simulink model "Controller"  (R2018b)
settings: configuration reference "control_config" (kept outside this file)
values from neighbouring files (symbols this model uses):
  CONTROL_EXPORT = Simulink.Parameter(CONTROL_EXPORT_VALUE)    [controller_model_init.m]
  CONTROL_PARAM = Simulink.Parameter(CONTROL_PARAM_VALUE)    [controller_model_init.m]
undefined symbols (not defined in the file or in its folder): actuator_cmd, CONTROL_CONST, CONTROL_PARAM_VALUE, ControlMode, DiscIntNeverNeededParam, PilotMode, timestamp
libraries: simulink x43, FMT_Model_Lib x6
(part 1 of 2)
settings Model: Creator=jc  LastModifiedBy=zouji
settings ConfigSetRef: SourceLocation=Base Workspace

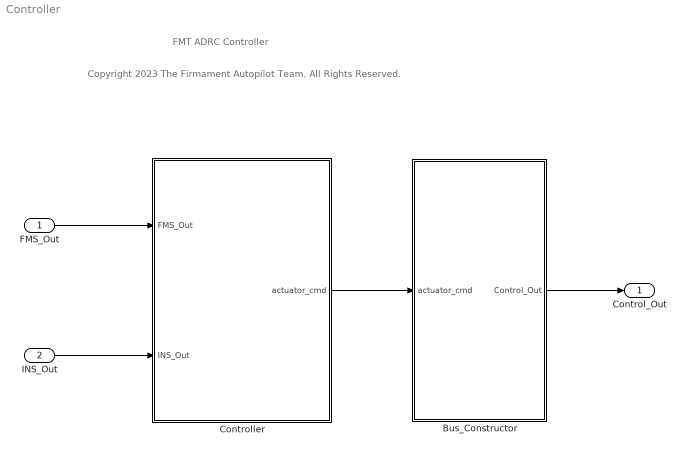
== system Controller ==
  note: Copyright 2023 The Firmament Autopilot Team. All Rights Reserved.
  note: FMT ADRC Controller
  FMS_Out : Inport  OutDataTypeStr=Bus: FMS_Out_Bus
  INS_Out : Inport  Port=2  OutDataTypeStr=Bus: INS_Out_Bus
  Bus_Constructor : Subsystem
  Controller : Subsystem
  Control_Out : Outport  OutDataTypeStr=Bus: Control_Out_Bus
  wires:
  FMS_Out/1 -> Controller/1(FMS_Out)
  INS_Out/1 -> Controller/2(INS_Out)
  Controller/1(actuator_cmd) -> Bus_Constructor/1(actuator_cmd)
  Bus_Constructor/1(Control_Out) -> Control_Out/1

== system Controller/Bus_Constructor ==
  actuator_cmd : Inport
  Bus Assignment : BusAssignment  AssignedSignals=actuator_cmd,timestamp
  Constant : Constant  Value=0  OutDataTypeStr=Bus: Control_Out_Bus
  timestamp : Subsystem  mask{sample_time=CONTROL_EXPORT.period}
      mask prompts: sample_time "sample time (ms)"
  Control_Out : Outport
  wires:
  actuator_cmd/1 -> Bus Assignment/2
  Constant/1 -> Bus Assignment/1
  Bus Assignment/1 -> Control_Out/1
  timestamp/1(timestamp_ms) -> Bus Assignment/3

== system Controller/Controller ==
  FMS_Out : Inport
  INS_Out : Inport  Port=2
  Control_Allocation : Subsystem  Variant=on
      settings: GeneratePreprocessorConditionals=on
  Horizontal_Control : Subsystem
  Vertical_Control : Subsystem
  actuator_cmd : Outport
  wires:
  FMS_Out/1 -> Control_Allocation/1(FMS_Out), Vertical_Control/1(FMS_Out), Horizontal_Control/1(FMS_Out)
  INS_Out/1 -> Horizontal_Control/2(INS_Out), Vertical_Control/2(INS_Out)
  Horizontal_Control/1(rate_dot_cmd_B) -> Control_Allocation/2(ang_acc_cmd)
  Vertical_Control/1(g_force_cmd_B) -> Control_Allocation/3(line_acc_cmd)
  Control_Allocation/1(actuator_cmd) -> actuator_cmd/1

== system Controller/Bus_Constructor/timestamp ==
  Constant : Constant  Value=sample_time
  Data Type Conversion : DataTypeConversion  OutDataTypeStr=uint32
  Discrete-Time Integrator : DiscreteIntegrator  IntegratorMethod=Accumulation: Forward Euler  SampleTime=-1  ICPrevOutput=DiscIntNeverNeededParam  ICPrevScaledInput=DiscIntNeverNeededParam
  timestamp_ms : Outport
  wires:
  Discrete-Time Integrator/1 -> Data Type Conversion/1
  Constant/1 -> Discrete-Time Integrator/1
  Data Type Conversion/1 -> timestamp_ms/1

== system Controller/Controller/Control_Allocation ==
  note: 1) Add Subsystem or Model blocks as valid variant choices.
      | 2) You cannot connect blocks at this level. At simulation, connectivity is automatically
      | determined, based on the active variant and port name matching.
  FMS_Out : Inport
  ang_acc_cmd : Inport  Port=2
  line_acc_cmd : Inport  Port=3
  Coxial_Hexacopter_x : Subsystem  TreatAsAtomicUnit=on  VariantControl=AIRFRAME==6
      mask Display: image('.\figures\cox_hexa_x.png');
  Coxial_Quadcopter_x : Subsystem  TreatAsAtomicUnit=on  VariantControl=AIRFRAME==3
      mask Display: image('.\figures\cox_quad_x.png');
  Hexacopter_+ : Subsystem  TreatAsAtomicUnit=on  VariantControl=AIRFRAME==5
      mask Display: image('.\figures\hexa_+.png');
  Hexacopter_x : Subsystem  TreatAsAtomicUnit=on  VariantControl=AIRFRAME==4
      mask Display: image('.\figures\hexa_x.png');
  Octocopter_+ : Subsystem  TreatAsAtomicUnit=on  VariantControl=AIRFRAME==8
      mask Display: image('.\figures\octo_+.png');
  Octocopter_x : Subsystem  TreatAsAtomicUnit=on  VariantControl=AIRFRAME==7
      mask Display: image('.\figures\octo_x.png');
  Quadcopter_+ : Subsystem  TreatAsAtomicUnit=on  VariantControl=AIRFRAME==2
      mask Display: image('.\figures\quad_+.png');
  Quadcopter_x : Subsystem  TreatAsAtomicUnit=on  VariantControl=AIRFRAME==1
      mask Display: image('.\figures\quad_x.png');
  actuator_cmd : Outport

== system Controller/Controller/Horizontal_Control ==
  FMS_Out : Inport
  INS_Out : Inport  Port=2
  Attitude_Controller : Subsystem
  Velocity_Controller : Subsystem
  rate_dot_cmd_B : Outport
  wires:
  Attitude_Controller/1(rate_dot_cmd_B) -> rate_dot_cmd_B/1
  FMS_Out/1 -> Attitude_Controller/2(FMS_Out), Velocity_Controller/1(FMS_Out)
  INS_Out/1 -> Velocity_Controller/2(INS_Out), Attitude_Controller/3(INS_Out)
  Velocity_Controller/1(att_cmd_B_rad) -> Attitude_Controller/1(att_cmd_B_rad)

== system Controller/Controller/Vertical_Control ==
  FMS_Out : Inport
  INS_Out : Inport  Port=2
  Veloxity_Z_Controller : Subsystem
  g_force_cmd_B : Outport
  wires:
  INS_Out/1 -> Veloxity_Z_Controller/2(INS_Out)
  Veloxity_Z_Controller/1(g_force_cmd_B) -> g_force_cmd_B/1
  FMS_Out/1 -> Veloxity_Z_Controller/1(FMS_Out)

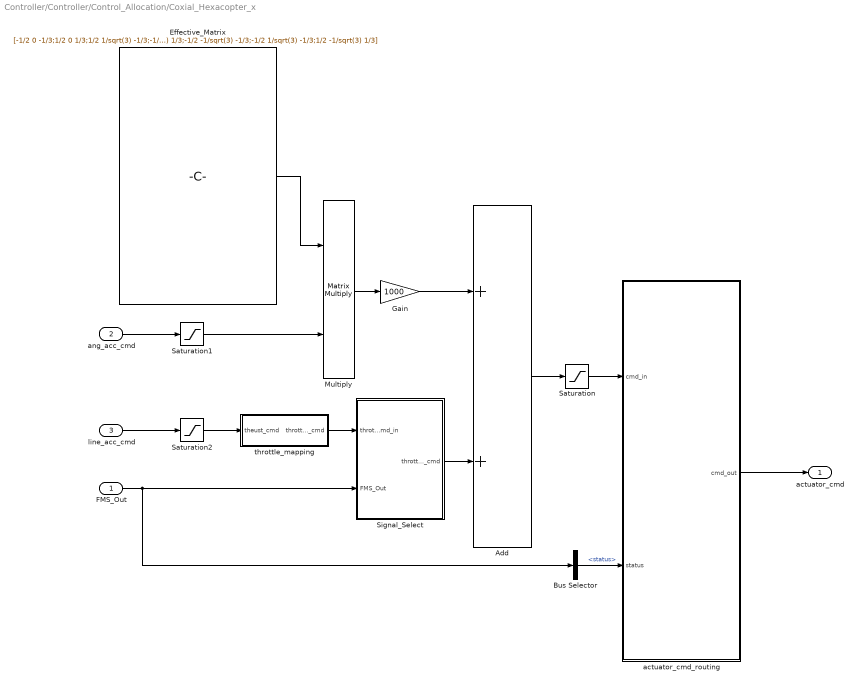
== system Controller/Controller/Control_Allocation/Coxial_Hexacopter_x ==
  FMS_Out : Inport
  ang_acc_cmd : Inport  Port=2
  line_acc_cmd : Inport  Port=3
  Add : Sum  OutDataTypeStr=uint16
  Bus Selector : BusSelector  OutputSignals=status
  Effective_Matrix : Constant  Value=[-1/2 0 -1/3;1/2 0 1/3;1/2 1/sqrt(3) -1/3;-1/2 -1/sqrt(3) 1/3;-1/2 1/sqrt(3) 1/3;1/2 -1/sqrt(3) -1/3;-1/2 0 1/3;1/2 0 -1/3;1/2 1/sqrt(3) 1/3;-1/2 -1/sqrt(3) -1/3;-1/2 1/sqrt(3) -1/3;1/2 -1/sqrt(3) 1/3]  OutDataTypeStr=single
  Gain : Gain  Gain=1000  OutDataTypeStr=uint16
  Multiply : Product  Multiplication=Matrix(*)  OutDataTypeStr=Inherit: Same as first input
  Saturation : Saturate  UpperLimit=1900  LowerLimit=1100
  Saturation1 : Saturate  UpperLimit=1  LowerLimit=-1
  Saturation2 : Saturate  UpperLimit=1  LowerLimit=-1
  Signal_Select : Subsystem
  actuator_cmd_routing : Subsystem
  throttle_mapping : Subsystem
  actuator_cmd : Outport
  wires:
  throttle_mapping/1(throttle_cmd) -> Signal_Select/1(throttle_cmd_in)
  Saturation2/1 -> throttle_mapping/1(theust_cmd)
  Gain/1 -> Add/1
  Multiply/1 -> Gain/1
  Signal_Select/1(throttle_cmd) -> Add/2
  Effective_Matrix/1 -> Multiply/1
  Saturation1/1 -> Multiply/2
  ang_acc_cmd/1 -> Saturation1/1
  line_acc_cmd/1 -> Saturation2/1
  actuator_cmd_routing/1(cmd_out) -> actuator_cmd/1
  Saturation/1 -> actuator_cmd_routing/1(cmd_in)
  FMS_Out/1 -> Bus Selector/1, Signal_Select/2(FMS_Out)
  Bus Selector/1 -> actuator_cmd_routing/2(status)  "<status>"
  Add/1 -> Saturation/1

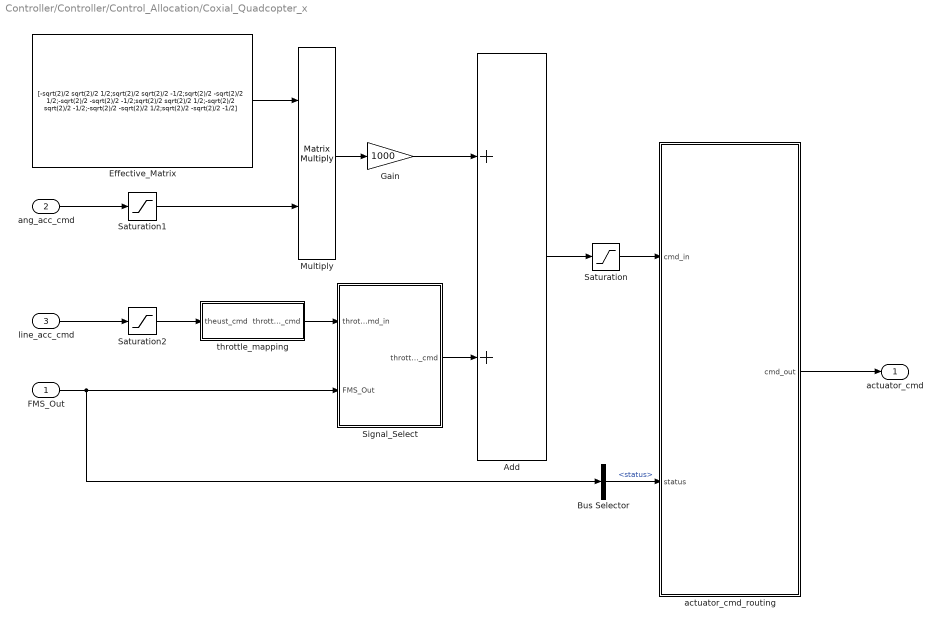
== system Controller/Controller/Control_Allocation/Coxial_Quadcopter_x ==
  FMS_Out : Inport
  ang_acc_cmd : Inport  Port=2
  line_acc_cmd : Inport  Port=3
  Add : Sum  OutDataTypeStr=uint16
  Bus Selector : BusSelector  OutputSignals=status
  Effective_Matrix : Constant  Value=[-sqrt(2)/2 sqrt(2)/2 1/2;sqrt(2)/2 sqrt(2)/2 -1/2;sqrt(2)/2 -sqrt(2)/2 1/2;-sqrt(2)/2 -sqrt(2)/2 -1/2;sqrt(2)/2 sqrt(2)/2 1/2;-sqrt(2)/2 sqrt(2)/2 -1/2;-sqrt(2)/2 -sqrt(2)/2 1/2;sqrt(2)/2 -sqrt(2)/2 -1/2]  OutDataTypeStr=single
  Gain : Gain  Gain=1000  OutDataTypeStr=uint16
  Multiply : Product  Multiplication=Matrix(*)  OutDataTypeStr=Inherit: Same as first input
  Saturation : Saturate  UpperLimit=1900  LowerLimit=1100
  Saturation1 : Saturate  UpperLimit=1  LowerLimit=-1
  Saturation2 : Saturate  UpperLimit=1  LowerLimit=-1
  Signal_Select : Subsystem
  actuator_cmd_routing : Subsystem
  throttle_mapping : Subsystem
  actuator_cmd : Outport
  wires:
  throttle_mapping/1(throttle_cmd) -> Signal_Select/1(throttle_cmd_in)
  Saturation2/1 -> throttle_mapping/1(theust_cmd)
  Gain/1 -> Add/1
  Multiply/1 -> Gain/1
  Signal_Select/1(throttle_cmd) -> Add/2
  Effective_Matrix/1 -> Multiply/1
  Saturation1/1 -> Multiply/2
  ang_acc_cmd/1 -> Saturation1/1
  line_acc_cmd/1 -> Saturation2/1
  actuator_cmd_routing/1(cmd_out) -> actuator_cmd/1
  Saturation/1 -> actuator_cmd_routing/1(cmd_in)
  FMS_Out/1 -> Bus Selector/1, Signal_Select/2(FMS_Out)
  Bus Selector/1 -> actuator_cmd_routing/2(status)  "<status>"
  Add/1 -> Saturation/1

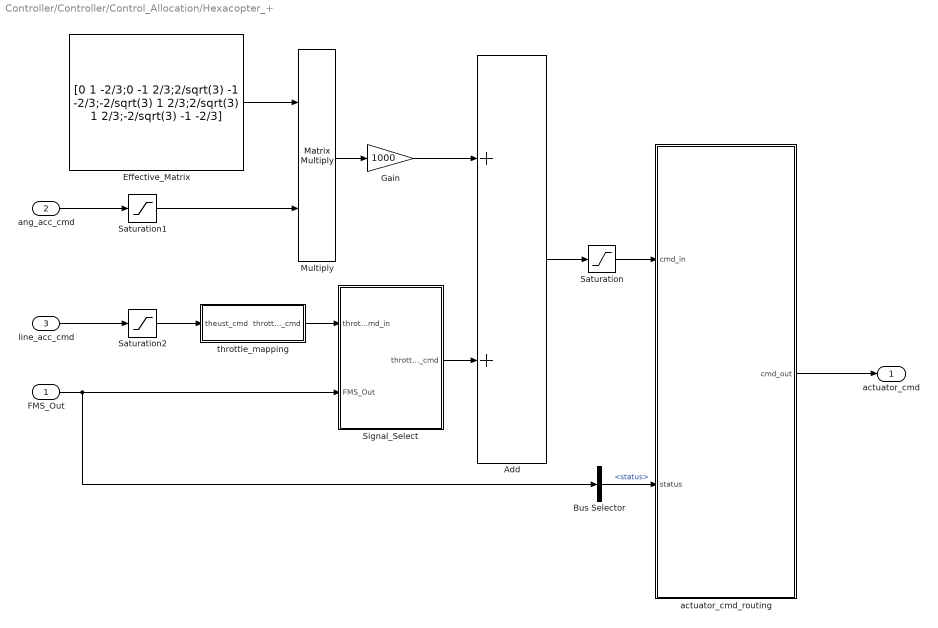
== system Controller/Controller/Control_Allocation/Hexacopter_+ ==
  FMS_Out : Inport
  ang_acc_cmd : Inport  Port=2
  line_acc_cmd : Inport  Port=3
  Add : Sum  OutDataTypeStr=uint16
  Bus Selector : BusSelector  OutputSignals=status
  Effective_Matrix : Constant  Value=[0 1 -2/3;0 -1 2/3;2/sqrt(3) -1 -2/3;-2/sqrt(3) 1 2/3;2/sqrt(3) 1 2/3;-2/sqrt(3) -1 -2/3]  OutDataTypeStr=single
  Gain : Gain  Gain=1000  OutDataTypeStr=uint16
  Multiply : Product  Multiplication=Matrix(*)  OutDataTypeStr=Inherit: Same as first input
  Saturation : Saturate  UpperLimit=1900  LowerLimit=1100
  Saturation1 : Saturate  UpperLimit=1  LowerLimit=-1
  Saturation2 : Saturate  UpperLimit=1  LowerLimit=-1
  Signal_Select : Subsystem
  actuator_cmd_routing : Subsystem
  throttle_mapping : Subsystem
  actuator_cmd : Outport
  wires:
  throttle_mapping/1(throttle_cmd) -> Signal_Select/1(throttle_cmd_in)
  Saturation2/1 -> throttle_mapping/1(theust_cmd)
  Gain/1 -> Add/1
  Multiply/1 -> Gain/1
  Signal_Select/1(throttle_cmd) -> Add/2
  Effective_Matrix/1 -> Multiply/1
  Saturation1/1 -> Multiply/2
  ang_acc_cmd/1 -> Saturation1/1
  line_acc_cmd/1 -> Saturation2/1
  actuator_cmd_routing/1(cmd_out) -> actuator_cmd/1
  Saturation/1 -> actuator_cmd_routing/1(cmd_in)
  FMS_Out/1 -> Bus Selector/1, Signal_Select/2(FMS_Out)
  Bus Selector/1 -> actuator_cmd_routing/2(status)  "<status>"
  Add/1 -> Saturation/1

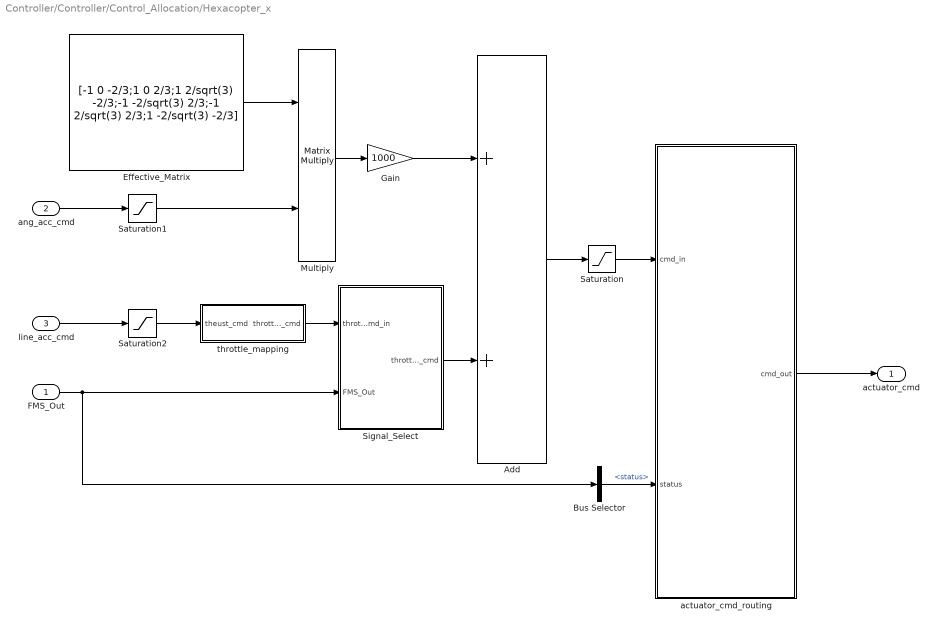
== system Controller/Controller/Control_Allocation/Hexacopter_x ==
  FMS_Out : Inport
  ang_acc_cmd : Inport  Port=2
  line_acc_cmd : Inport  Port=3
  Add : Sum  OutDataTypeStr=uint16
  Bus Selector : BusSelector  OutputSignals=status
  Effective_Matrix : Constant  Value=[-1 0 -2/3;1 0 2/3;1 2/sqrt(3) -2/3;-1 -2/sqrt(3) 2/3;-1 2/sqrt(3) 2/3;1 -2/sqrt(3) -2/3]  OutDataTypeStr=single
  Gain : Gain  Gain=1000  OutDataTypeStr=uint16
  Multiply : Product  Multiplication=Matrix(*)  OutDataTypeStr=Inherit: Same as first input
  Saturation : Saturate  UpperLimit=1900  LowerLimit=1100
  Saturation1 : Saturate  UpperLimit=1  LowerLimit=-1
  Saturation2 : Saturate  UpperLimit=1  LowerLimit=-1
  Signal_Select : Subsystem
  actuator_cmd_routing : Subsystem
  throttle_mapping : Subsystem
  actuator_cmd : Outport
  wires:
  throttle_mapping/1(throttle_cmd) -> Signal_Select/1(throttle_cmd_in)
  Saturation2/1 -> throttle_mapping/1(theust_cmd)
  Gain/1 -> Add/1
  Multiply/1 -> Gain/1
  Signal_Select/1(throttle_cmd) -> Add/2
  Effective_Matrix/1 -> Multiply/1
  Saturation1/1 -> Multiply/2
  ang_acc_cmd/1 -> Saturation1/1
  line_acc_cmd/1 -> Saturation2/1
  actuator_cmd_routing/1(cmd_out) -> actuator_cmd/1
  Saturation/1 -> actuator_cmd_routing/1(cmd_in)
  FMS_Out/1 -> Bus Selector/1, Signal_Select/2(FMS_Out)
  Bus Selector/1 -> actuator_cmd_routing/2(status)  "<status>"
  Add/1 -> Saturation/1

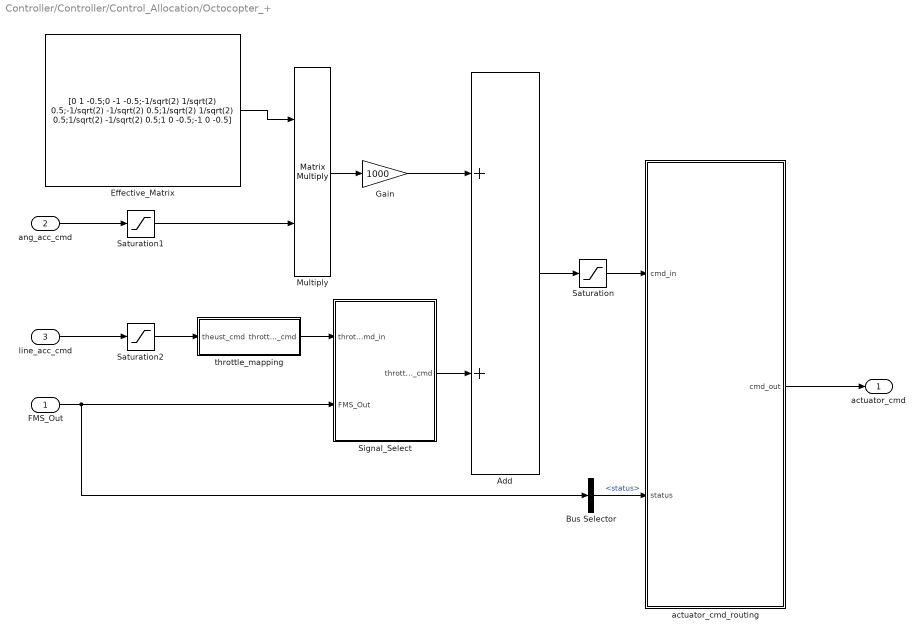
== system Controller/Controller/Control_Allocation/Octocopter_+ ==
  FMS_Out : Inport
  ang_acc_cmd : Inport  Port=2
  line_acc_cmd : Inport  Port=3
  Add : Sum  OutDataTypeStr=uint16
  Bus Selector : BusSelector  OutputSignals=status
  Effective_Matrix : Constant  Value=[0 1 -0.5;0 -1 -0.5;-1/sqrt(2) 1/sqrt(2) 0.5;-1/sqrt(2) -1/sqrt(2) 0.5;1/sqrt(2) 1/sqrt(2) 0.5;1/sqrt(2) -1/sqrt(2) 0.5;1 0 -0.5;-1 0 -0.5]  OutDataTypeStr=single
  Gain : Gain  Gain=1000  OutDataTypeStr=uint16
  Multiply : Product  Multiplication=Matrix(*)  OutDataTypeStr=Inherit: Same as first input
  Saturation : Saturate  UpperLimit=1900  LowerLimit=1100
  Saturation1 : Saturate  UpperLimit=1  LowerLimit=-1
  Saturation2 : Saturate  UpperLimit=1  LowerLimit=-1
  Signal_Select : Subsystem
  actuator_cmd_routing : Subsystem
  throttle_mapping : Subsystem
  actuator_cmd : Outport
  wires:
  throttle_mapping/1(throttle_cmd) -> Signal_Select/1(throttle_cmd_in)
  Saturation2/1 -> throttle_mapping/1(theust_cmd)
  Gain/1 -> Add/1
  Multiply/1 -> Gain/1
  Signal_Select/1(throttle_cmd) -> Add/2
  Effective_Matrix/1 -> Multiply/1
  Saturation1/1 -> Multiply/2
  ang_acc_cmd/1 -> Saturation1/1
  line_acc_cmd/1 -> Saturation2/1
  actuator_cmd_routing/1(cmd_out) -> actuator_cmd/1
  Saturation/1 -> actuator_cmd_routing/1(cmd_in)
  FMS_Out/1 -> Bus Selector/1, Signal_Select/2(FMS_Out)
  Bus Selector/1 -> actuator_cmd_routing/2(status)  "<status>"
  Add/1 -> Saturation/1

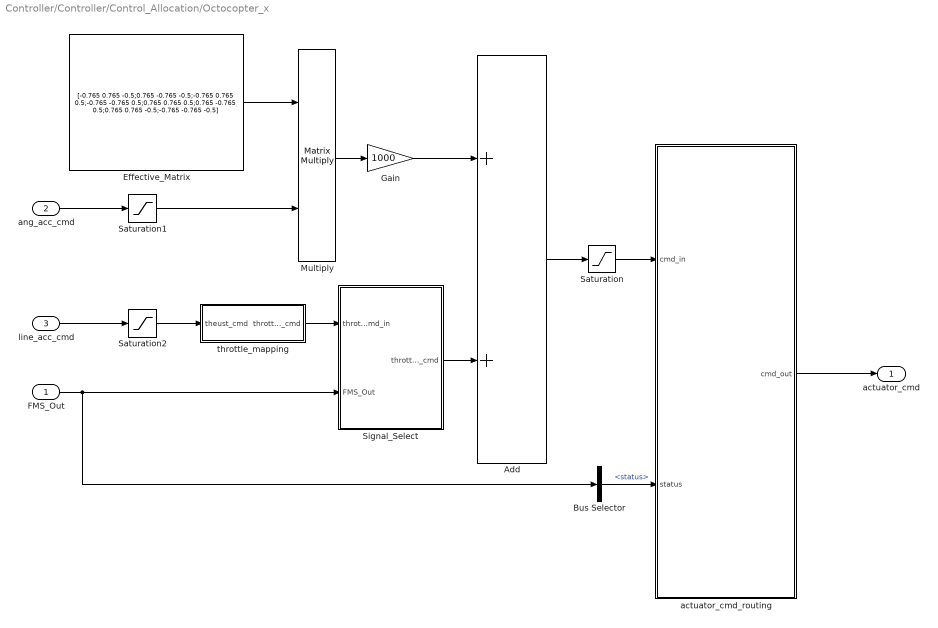
== system Controller/Controller/Control_Allocation/Octocopter_x ==
  FMS_Out : Inport
  ang_acc_cmd : Inport  Port=2
  line_acc_cmd : Inport  Port=3
  Add : Sum  OutDataTypeStr=uint16
  Bus Selector : BusSelector  OutputSignals=status
  Effective_Matrix : Constant  Value=[-0.765 0.765 -0.5;0.765 -0.765 -0.5;-0.765 0.765 0.5;-0.765 -0.765 0.5;0.765 0.765 0.5;0.765 -0.765 0.5;0.765 0.765 -0.5;-0.765 -0.765 -0.5]  OutDataTypeStr=single
  Gain : Gain  Gain=1000  OutDataTypeStr=uint16
  Multiply : Product  Multiplication=Matrix(*)  OutDataTypeStr=Inherit: Same as first input
  Saturation : Saturate  UpperLimit=1900  LowerLimit=1100
  Saturation1 : Saturate  UpperLimit=1  LowerLimit=-1
  Saturation2 : Saturate  UpperLimit=1  LowerLimit=-1
  Signal_Select : Subsystem
  actuator_cmd_routing : Subsystem
  throttle_mapping : Subsystem
  actuator_cmd : Outport
  wires:
  throttle_mapping/1(throttle_cmd) -> Signal_Select/1(throttle_cmd_in)
  Saturation2/1 -> throttle_mapping/1(theust_cmd)
  Gain/1 -> Add/1
  Multiply/1 -> Gain/1
  Signal_Select/1(throttle_cmd) -> Add/2
  Effective_Matrix/1 -> Multiply/1
  Saturation1/1 -> Multiply/2
  ang_acc_cmd/1 -> Saturation1/1
  line_acc_cmd/1 -> Saturation2/1
  actuator_cmd_routing/1(cmd_out) -> actuator_cmd/1
  Saturation/1 -> actuator_cmd_routing/1(cmd_in)
  FMS_Out/1 -> Bus Selector/1, Signal_Select/2(FMS_Out)
  Bus Selector/1 -> actuator_cmd_routing/2(status)  "<status>"
  Add/1 -> Saturation/1

== system Controller/Controller/Control_Allocation/Quadcopter_+ ==
  FMS_Out : Inport
  ang_acc_cmd : Inport  Port=2
  line_acc_cmd : Inport  Port=3
  Add : Sum  OutDataTypeStr=uint16
  Bus Selector : BusSelector  OutputSignals=status
  Effective_Matrix : Constant  Value=[-2 0 1;2 0 1;0 2 -1;0 -2 -1]  OutDataTypeStr=single
  Gain : Gain  Gain=1000  OutDataTypeStr=uint16
  Multiply : Product  Multiplication=Matrix(*)  OutDataTypeStr=Inherit: Same as first input
  Saturation : Saturate  UpperLimit=1900  LowerLimit=1100
  Saturation1 : Saturate  UpperLimit=1  LowerLimit=-1
  Saturation2 : Saturate  UpperLimit=1  LowerLimit=-1
  Signal_Select : Subsystem
  actuator_cmd_routing : Subsystem
  throttle_mapping : Subsystem
  actuator_cmd : Outport
  wires:
  throttle_mapping/1(throttle_cmd) -> Signal_Select/1(throttle_cmd_in)
  Saturation2/1 -> throttle_mapping/1(theust_cmd)
  Gain/1 -> Add/1
  Multiply/1 -> Gain/1
  Signal_Select/1(throttle_cmd) -> Add/2
  Effective_Matrix/1 -> Multiply/1
  Saturation1/1 -> Multiply/2
  ang_acc_cmd/1 -> Saturation1/1
  line_acc_cmd/1 -> Saturation2/1
  actuator_cmd_routing/1(cmd_out) -> actuator_cmd/1
  Saturation/1 -> actuator_cmd_routing/1(cmd_in)
  FMS_Out/1 -> Bus Selector/1, Signal_Select/2(FMS_Out)
  Bus Selector/1 -> actuator_cmd_routing/2(status)  "<status>"
  Add/1 -> Saturation/1

== system Controller/Controller/Control_Allocation/Quadcopter_x ==
  FMS_Out : Inport
  ang_acc_cmd : Inport  Port=2
  line_acc_cmd : Inport  Port=3
  Add : Sum  OutDataTypeStr=uint16
  Bus Selector : BusSelector  OutputSignals=status
  Effective_Matrix : Constant  Value=[-sqrt(2) sqrt(2) 1;sqrt(2) -sqrt(2) 1;sqrt(2) sqrt(2) -1;-sqrt(2) -sqrt(2) -1]  OutDataTypeStr=single
  Gain : Gain  Gain=1000  OutDataTypeStr=uint16
  Multiply : Product  Multiplication=Matrix(*)  OutDataTypeStr=Inherit: Same as first input
  Saturation : Saturate  UpperLimit=1900  LowerLimit=1100
  Saturation1 : Saturate  UpperLimit=1  LowerLimit=-1
  Saturation2 : Saturate  UpperLimit=1  LowerLimit=-1
  Signal_Select : Subsystem
  actuator_cmd_routing : Subsystem
  throttle_mapping : Subsystem
  actuator_cmd : Outport
  wires:
  throttle_mapping/1(throttle_cmd) -> Signal_Select/1(throttle_cmd_in)
  Saturation2/1 -> throttle_mapping/1(theust_cmd)
  Add/1 -> Saturation/1
  Gain/1 -> Add/1
  Multiply/1 -> Gain/1
  FMS_Out/1 -> Bus Selector/1, Signal_Select/2(FMS_Out)
  Signal_Select/1(throttle_cmd) -> Add/2
  Effective_Matrix/1 -> Multiply/1
  Saturation1/1 -> Multiply/2
  ang_acc_cmd/1 -> Saturation1/1
  line_acc_cmd/1 -> Saturation2/1
  actuator_cmd_routing/1(cmd_out) -> actuator_cmd/1
  Saturation/1 -> actuator_cmd_routing/1(cmd_in)
  Bus Selector/1 -> actuator_cmd_routing/2(status)  "<status>"

== system Controller/Controller/Horizontal_Control/Attitude_Controller ==
  att_cmd_B_rad : Inport
  FMS_Out : Inport  Port=2
  INS_Out : Inport  Port=3
  Inner_Loop : Subsystem
  Outter_Loop : Subsystem
  rate_dot_cmd_B : Outport
  wires:
  INS_Out/1 -> Inner_Loop/2(INS_Out), Outter_Loop/2(INS_Out)
  FMS_Out/1 -> Inner_Loop/3(FMS_Out), Outter_Loop/3(FMS_Out)
  att_cmd_B_rad/1 -> Outter_Loop/1(att_cmd_rad)
  Outter_Loop/1(euler_rate_cmd_radPs) -> Inner_Loop/1(euler_rate_cmd_radPs)
  Inner_Loop/1(rate_dot_cmd_B) -> rate_dot_cmd_B/1

== system Controller/Controller/Horizontal_Control/Velocity_Controller ==
  FMS_Out : Inport
  INS_Out : Inport  Port=2
  Accel_to_Attitude_CMD : Subsystem
  Bus Selector : BusSelector  OutputSignals=reset
  Error : Subsystem
  PID_Controller : Subsystem
  Signal_Select : Subsystem
  att_cmd_B_rad : Outport
  wires:
  FMS_Out/1 -> Error/2(FMS_Out), Signal_Select/2(FMS_Out), Bus Selector/1
  PID_Controller/1(accel_cmd_C) -> Signal_Select/1(acc_cmd_in)  "accel_cmd_C_mPs2"
  INS_Out/1 -> Error/1(INS_Out)
  Error/1(uv_err_C_mPs) -> PID_Controller/1(uv_err_C_mPs)
  Accel_to_Attitude_CMD/1(att_cmd_B_rad) -> att_cmd_B_rad/1
  Bus Selector/1 -> PID_Controller/2(reset)  "<reset>"
  Signal_Select/1(acc_cmd_out) -> Accel_to_Attitude_CMD/1(accel_cmd_C_mPs2)

== system Controller/Controller/Vertical_Control/Veloxity_Z_Controller ==
  note: Leave some margin
      | for att control
  FMS_Out : Inport
  INS_Out : Inport  Port=2
  Boosted_Throttle : Subsystem
  Bus Selector : BusSelector  OutputSignals=reset
  Error : Subsystem
  PID_Controller : Subsystem
  Saturation : Saturate  UpperLimit=0.35  LowerLimit=-0.35
  g_force_cmd_B : Outport
  wires:
  Saturation/1 -> g_force_cmd_B/1
  FMS_Out/1 -> Error/1(FMS_Out), Bus Selector/1
  INS_Out/1 -> Error/2(INS_Out), Boosted_Throttle/2(INS_Out)
  Boosted_Throttle/1(boosted_thrust) -> Saturation/1  "boosted_thrust"
  Error/1(az_cmd_C_mPs2) -> PID_Controller/1(az_cmd_C_mPs2)
  Bus Selector/1 -> PID_Controller/2(reset)  "<reset>"
  PID_Controller/1(thrust_cmd) -> Boosted_Throttle/1(thrust_cmd)

== system Controller/Controller/Control_Allocation/Coxial_Hexacopter_x/Signal_Select ==
  note: mode:
      | 0: Unknown
      | 1: Mission
      | 2: Position
      | 3: Altitude Hold
      | 4: Manual Mode
      | 5: Acro Mode
  throttle_cmd_in : Inport
  FMS_Out : Inport  Port=2
  Bus Selector1 : BusSelector  OutputSignals=throttle_cmd,ctrl_mode
  Compare To Constant : simulink/Logic and Bit Operations/Compare To Constant  relop===  const=uint8([ControlMode.Manual, ControlMode.Acro, ControlMode.Stabilize])  OutDataTypeStr=boolean
  Compare To Constant1 : simulink/Logic and Bit Operations/Compare To Constant  relop===  const=uint8(ControlMode.Offboard)  OutDataTypeStr=boolean
  Logical Operator : Logic  Operator=OR  Inputs=1  AllPortsSameDT=off  OutDataTypeStr=boolean
  Offboard_Signal_Select : Subsystem
  Switch : Switch  Criteria=u2 > Threshold
  Switch1 : Switch  Criteria=u2 > Threshold
  throttle_cmd : Outport
  wires:
  Compare To Constant/1 -> Logical Operator/1
  FMS_Out/1 -> Offboard_Signal_Select/1(FMS_Out), Bus Selector1/1
  Bus Selector1/1 -> Switch/1  "<throttle_cmd>"
  Bus Selector1/2 -> Compare To Constant1/1, Compare To Constant/1  "<ctrl_mode>"
  Switch/1 -> throttle_cmd/1  "throttle_cmd"
  Logical Operator/1 -> Switch/2
  throttle_cmd_in/1 -> Offboard_Signal_Select/2(throttle_cmd_in), Switch1/3
  Compare To Constant1/1 -> Switch1/2
  Switch1/1 -> Switch/3
  Offboard_Signal_Select/1(throttle_cmd_out) -> Switch1/1

== system Controller/Controller/Control_Allocation/Coxial_Hexacopter_x/actuator_cmd_routing ==
  cmd_in : Inport
  status : Inport  Port=2
  Constant : Constant  Value=zeros(4,1)  VectorParams1D=off  OutDataTypeStr=uint16
  Disarm : Constant  Value=ones(12,1)*1000  VectorParams1D=off  OutDataTypeStr=uint16
  Multiport Switch : MultiPortSwitch  DataPortForDefault=Additional data port  DiagnosticForDefault=None
  Mux1 : Mux  Inputs=2
  Reshape : Reshape  OutputDimensionality=Customize  OutputDimensions=[16,1]
  Standby : Constant  Value=ones(12,1)*1150  VectorParams1D=off  OutDataTypeStr=uint16
  cmd_out : Outport
  wires:
  Disarm/1 -> Multiport Switch/5, Multiport Switch/2
  Reshape/1 -> cmd_out/1
  Constant/1 -> Mux1/2
  Standby/1 -> Multiport Switch/3
  Mux1/1 -> Reshape/1
  status/1 -> Multiport Switch/1
  Multiport Switch/1 -> Mux1/1
  cmd_in/1 -> Multiport Switch/4

== system Controller/Controller/Control_Allocation/Coxial_Hexacopter_x/throttle_mapping ==
  theust_cmd : Inport
  Constant1 : Constant  Value=1000  OutDataTypeStr=uint32
  Data Type Conversion : DataTypeConversion  OutDataTypeStr=uint16
  Gain1 : Gain  Gain=1000  OutDataTypeStr=uint32
  Saturation : Saturate  UpperLimit=1  LowerLimit=0
  Sum : Sum  Inputs=|++
  Sum1 : Sum  Inputs=|++
  hover_throttle : Constant  Value=CONTROL_PARAM.HOVER_THRO  OutDataTypeStr=Inherit: Inherit via back propagation
  throttle_cmd : Outport
  wires:
  theust_cmd/1 -> Sum/1
  Sum/1 -> Saturation/1
  hover_throttle/1 -> Sum/2
  Gain1/1 -> Sum1/1
  Constant1/1 -> Sum1/2
  Data Type Conversion/1 -> throttle_cmd/1
  Saturation/1 -> Gain1/1
  Sum1/1 -> Data Type Conversion/1

== system Controller/Controller/Control_Allocation/Coxial_Quadcopter_x/Signal_Select ==
  note: mode:
      | 0: Unknown
      | 1: Mission
      | 2: Position
      | 3: Altitude Hold
      | 4: Manual Mode
      | 5: Acro Mode
  throttle_cmd_in : Inport
  FMS_Out : Inport  Port=2
  Bus Selector1 : BusSelector  OutputSignals=throttle_cmd,ctrl_mode
  Compare To Constant : simulink/Logic and Bit Operations/Compare To Constant  relop===  const=uint8([ControlMode.Manual, ControlMode.Acro, ControlMode.Stabilize])  OutDataTypeStr=boolean
  Compare To Constant1 : simulink/Logic and Bit Operations/Compare To Constant  relop===  const=uint8(ControlMode.Offboard)  OutDataTypeStr=boolean
  Logical Operator : Logic  Operator=OR  Inputs=1  AllPortsSameDT=off  OutDataTypeStr=boolean
  Offboard_Signal_Select : Subsystem
  Switch : Switch  Criteria=u2 > Threshold
  Switch1 : Switch  Criteria=u2 > Threshold
  throttle_cmd : Outport
  wires:
  Compare To Constant/1 -> Logical Operator/1
  FMS_Out/1 -> Offboard_Signal_Select/1(FMS_Out), Bus Selector1/1
  Bus Selector1/1 -> Switch/1  "<throttle_cmd>"
  Bus Selector1/2 -> Compare To Constant1/1, Compare To Constant/1  "<ctrl_mode>"
  Switch/1 -> throttle_cmd/1  "throttle_cmd"
  Logical Operator/1 -> Switch/2
  throttle_cmd_in/1 -> Offboard_Signal_Select/2(throttle_cmd_in), Switch1/3
  Compare To Constant1/1 -> Switch1/2
  Switch1/1 -> Switch/3
  Offboard_Signal_Select/1(throttle_cmd_out) -> Switch1/1

== system Controller/Controller/Control_Allocation/Coxial_Quadcopter_x/actuator_cmd_routing ==
  cmd_in : Inport
  status : Inport  Port=2
  Constant : Constant  Value=zeros(8,1)  VectorParams1D=off  OutDataTypeStr=uint16
  Disarm : Constant  Value=ones(8,1)*1000  VectorParams1D=off  OutDataTypeStr=uint16
  Multiport Switch : MultiPortSwitch  DataPortForDefault=Additional data port  DiagnosticForDefault=None
  Mux1 : Mux  Inputs=2
  Reshape : Reshape  OutputDimensionality=Customize  OutputDimensions=[16,1]
  Standby : Constant  Value=ones(8,1)*1150  VectorParams1D=off  OutDataTypeStr=uint16
  cmd_out : Outport
  wires:
  Disarm/1 -> Multiport Switch/5, Multiport Switch/2
  Reshape/1 -> cmd_out/1
  Constant/1 -> Mux1/2
  Standby/1 -> Multiport Switch/3
  Mux1/1 -> Reshape/1
  status/1 -> Multiport Switch/1
  Multiport Switch/1 -> Mux1/1
  cmd_in/1 -> Multiport Switch/4

== system Controller/Controller/Control_Allocation/Coxial_Quadcopter_x/throttle_mapping ==
  theust_cmd : Inport
  Constant1 : Constant  Value=1000  OutDataTypeStr=uint32
  Data Type Conversion : DataTypeConversion  OutDataTypeStr=uint16
  Gain1 : Gain  Gain=1000  OutDataTypeStr=uint32
  Saturation : Saturate  UpperLimit=1  LowerLimit=0
  Sum : Sum  Inputs=|++
  Sum1 : Sum  Inputs=|++
  hover_throttle : Constant  Value=CONTROL_PARAM.HOVER_THRO  OutDataTypeStr=Inherit: Inherit via back propagation
  throttle_cmd : Outport
  wires:
  theust_cmd/1 -> Sum/1
  Sum/1 -> Saturation/1
  hover_throttle/1 -> Sum/2
  Gain1/1 -> Sum1/1
  Constant1/1 -> Sum1/2
  Data Type Conversion/1 -> throttle_cmd/1
  Saturation/1 -> Gain1/1
  Sum1/1 -> Data Type Conversion/1

== system Controller/Controller/Control_Allocation/Hexacopter_+/Signal_Select ==
  note: mode:
      | 0: Unknown
      | 1: Mission
      | 2: Position
      | 3: Altitude Hold
      | 4: Manual Mode
      | 5: Acro Mode
  throttle_cmd_in : Inport
  FMS_Out : Inport  Port=2
  Bus Selector1 : BusSelector  OutputSignals=throttle_cmd,ctrl_mode
  Compare To Constant : simulink/Logic and Bit Operations/Compare To Constant  relop===  const=uint8([ControlMode.Manual, ControlMode.Acro, ControlMode.Stabilize])  OutDataTypeStr=boolean
  Compare To Constant1 : simulink/Logic and Bit Operations/Compare To Constant  relop===  const=uint8(ControlMode.Offboard)  OutDataTypeStr=boolean
  Logical Operator : Logic  Operator=OR  Inputs=1  AllPortsSameDT=off  OutDataTypeStr=boolean
  Offboard_Signal_Select : Subsystem
  Switch : Switch  Criteria=u2 > Threshold
  Switch1 : Switch  Criteria=u2 > Threshold
  throttle_cmd : Outport
  wires:
  Compare To Constant/1 -> Logical Operator/1
  FMS_Out/1 -> Offboard_Signal_Select/1(FMS_Out), Bus Selector1/1
  Bus Selector1/1 -> Switch/1  "<throttle_cmd>"
  Bus Selector1/2 -> Compare To Constant1/1, Compare To Constant/1  "<ctrl_mode>"
  Switch/1 -> throttle_cmd/1  "throttle_cmd"
  Logical Operator/1 -> Switch/2
  throttle_cmd_in/1 -> Offboard_Signal_Select/2(throttle_cmd_in), Switch1/3
  Compare To Constant1/1 -> Switch1/2
  Switch1/1 -> Switch/3
  Offboard_Signal_Select/1(throttle_cmd_out) -> Switch1/1

== system Controller/Controller/Control_Allocation/Hexacopter_+/actuator_cmd_routing ==
  cmd_in : Inport
  status : Inport  Port=2
  Constant : Constant  Value=zeros(10,1)  VectorParams1D=off  OutDataTypeStr=uint16
  Disarm : Constant  Value=ones(6,1)*1000  VectorParams1D=off  OutDataTypeStr=uint16
  Multiport Switch : MultiPortSwitch  DataPortForDefault=Additional data port  DiagnosticForDefault=None
  Mux1 : Mux  Inputs=2
  Reshape : Reshape  OutputDimensionality=Customize  OutputDimensions=[16,1]
  Standby : Constant  Value=ones(6,1)*1150  VectorParams1D=off  OutDataTypeStr=uint16
  cmd_out : Outport
  wires:
  Disarm/1 -> Multiport Switch/5, Multiport Switch/2
  Reshape/1 -> cmd_out/1
  Constant/1 -> Mux1/2
  Standby/1 -> Multiport Switch/3
  Mux1/1 -> Reshape/1
  status/1 -> Multiport Switch/1
  Multiport Switch/1 -> Mux1/1
  cmd_in/1 -> Multiport Switch/4

== system Controller/Controller/Control_Allocation/Hexacopter_+/throttle_mapping ==
  theust_cmd : Inport
  Constant1 : Constant  Value=1000  OutDataTypeStr=uint32
  Data Type Conversion : DataTypeConversion  OutDataTypeStr=uint16
  Gain1 : Gain  Gain=1000  OutDataTypeStr=uint32
  Saturation : Saturate  UpperLimit=1  LowerLimit=0
  Sum : Sum  Inputs=|++
  Sum1 : Sum  Inputs=|++
  hover_throttle : Constant  Value=CONTROL_PARAM.HOVER_THRO  OutDataTypeStr=Inherit: Inherit via back propagation
  throttle_cmd : Outport
  wires:
  theust_cmd/1 -> Sum/1
  Sum/1 -> Saturation/1
  hover_throttle/1 -> Sum/2
  Gain1/1 -> Sum1/1
  Constant1/1 -> Sum1/2
  Data Type Conversion/1 -> throttle_cmd/1
  Saturation/1 -> Gain1/1
  Sum1/1 -> Data Type Conversion/1

== system Controller/Controller/Control_Allocation/Hexacopter_x/Signal_Select ==
  note: mode:
      | 0: Unknown
      | 1: Mission
      | 2: Position
      | 3: Altitude Hold
      | 4: Manual Mode
      | 5: Acro Mode
  throttle_cmd_in : Inport
  FMS_Out : Inport  Port=2
  Bus Selector1 : BusSelector  OutputSignals=throttle_cmd,ctrl_mode
  Compare To Constant : simulink/Logic and Bit Operations/Compare To Constant  relop===  const=uint8([ControlMode.Manual, ControlMode.Acro, ControlMode.Stabilize])  OutDataTypeStr=boolean
  Compare To Constant1 : simulink/Logic and Bit Operations/Compare To Constant  relop===  const=uint8(ControlMode.Offboard)  OutDataTypeStr=boolean
  Logical Operator : Logic  Operator=OR  Inputs=1  AllPortsSameDT=off  OutDataTypeStr=boolean
  Offboard_Signal_Select : Subsystem
  Switch : Switch  Criteria=u2 > Threshold
  Switch1 : Switch  Criteria=u2 > Threshold
  throttle_cmd : Outport
  wires:
  Compare To Constant/1 -> Logical Operator/1
  FMS_Out/1 -> Offboard_Signal_Select/1(FMS_Out), Bus Selector1/1
  Bus Selector1/1 -> Switch/1  "<throttle_cmd>"
  Bus Selector1/2 -> Compare To Constant1/1, Compare To Constant/1  "<ctrl_mode>"
  Switch/1 -> throttle_cmd/1  "throttle_cmd"
  Logical Operator/1 -> Switch/2
  throttle_cmd_in/1 -> Offboard_Signal_Select/2(throttle_cmd_in), Switch1/3
  Compare To Constant1/1 -> Switch1/2
  Switch1/1 -> Switch/3
  Offboard_Signal_Select/1(throttle_cmd_out) -> Switch1/1

== system Controller/Controller/Control_Allocation/Hexacopter_x/actuator_cmd_routing ==
  cmd_in : Inport
  status : Inport  Port=2
  Constant : Constant  Value=zeros(10,1)  VectorParams1D=off  OutDataTypeStr=uint16
  Disarm : Constant  Value=ones(6,1)*1000  VectorParams1D=off  OutDataTypeStr=uint16
  Multiport Switch : MultiPortSwitch  DataPortForDefault=Additional data port  DiagnosticForDefault=None
  Mux1 : Mux  Inputs=2
  Reshape : Reshape  OutputDimensionality=Customize  OutputDimensions=[16,1]
  Standby : Constant  Value=ones(6,1)*1150  VectorParams1D=off  OutDataTypeStr=uint16
  cmd_out : Outport
  wires:
  Disarm/1 -> Multiport Switch/5, Multiport Switch/2
  Reshape/1 -> cmd_out/1
  Constant/1 -> Mux1/2
  Standby/1 -> Multiport Switch/3
  Mux1/1 -> Reshape/1
  status/1 -> Multiport Switch/1
  Multiport Switch/1 -> Mux1/1
  cmd_in/1 -> Multiport Switch/4

== system Controller/Controller/Control_Allocation/Hexacopter_x/throttle_mapping ==
  theust_cmd : Inport
  Constant1 : Constant  Value=1000  OutDataTypeStr=uint32
  Data Type Conversion : DataTypeConversion  OutDataTypeStr=uint16
  Gain1 : Gain  Gain=1000  OutDataTypeStr=uint32
  Saturation : Saturate  UpperLimit=1  LowerLimit=0
  Sum : Sum  Inputs=|++
  Sum1 : Sum  Inputs=|++
  hover_throttle : Constant  Value=CONTROL_PARAM.HOVER_THRO  OutDataTypeStr=Inherit: Inherit via back propagation
  throttle_cmd : Outport
  wires:
  theust_cmd/1 -> Sum/1
  Sum/1 -> Saturation/1
  hover_throttle/1 -> Sum/2
  Gain1/1 -> Sum1/1
  Constant1/1 -> Sum1/2
  Data Type Conversion/1 -> throttle_cmd/1
  Saturation/1 -> Gain1/1
  Sum1/1 -> Data Type Conversion/1

== system Controller/Controller/Control_Allocation/Octocopter_+/Signal_Select ==
  note: mode:
      | 0: Unknown
      | 1: Mission
      | 2: Position
      | 3: Altitude Hold
      | 4: Manual Mode
      | 5: Acro Mode
  throttle_cmd_in : Inport
  FMS_Out : Inport  Port=2
  Bus Selector1 : BusSelector  OutputSignals=throttle_cmd,ctrl_mode
  Compare To Constant : simulink/Logic and Bit Operations/Compare To Constant  relop===  const=uint8([ControlMode.Manual, ControlMode.Acro, ControlMode.Stabilize])  OutDataTypeStr=boolean
  Compare To Constant1 : simulink/Logic and Bit Operations/Compare To Constant  relop===  const=uint8(ControlMode.Offboard)  OutDataTypeStr=boolean
  Logical Operator : Logic  Operator=OR  Inputs=1  AllPortsSameDT=off  OutDataTypeStr=boolean
  Offboard_Signal_Select : Subsystem
  Switch : Switch  Criteria=u2 > Threshold
  Switch1 : Switch  Criteria=u2 > Threshold
  throttle_cmd : Outport
  wires:
  Compare To Constant/1 -> Logical Operator/1
  FMS_Out/1 -> Offboard_Signal_Select/1(FMS_Out), Bus Selector1/1
  Bus Selector1/1 -> Switch/1  "<throttle_cmd>"
  Bus Selector1/2 -> Compare To Constant1/1, Compare To Constant/1  "<ctrl_mode>"
  Switch/1 -> throttle_cmd/1  "throttle_cmd"
  Logical Operator/1 -> Switch/2
  throttle_cmd_in/1 -> Offboard_Signal_Select/2(throttle_cmd_in), Switch1/3
  Compare To Constant1/1 -> Switch1/2
  Switch1/1 -> Switch/3
  Offboard_Signal_Select/1(throttle_cmd_out) -> Switch1/1

== system Controller/Controller/Control_Allocation/Octocopter_+/actuator_cmd_routing ==
  cmd_in : Inport
  status : Inport  Port=2
  Constant : Constant  Value=zeros(8,1)  VectorParams1D=off  OutDataTypeStr=uint16
  Disarm : Constant  Value=ones(8,1)*1000  VectorParams1D=off  OutDataTypeStr=uint16
  Multiport Switch : MultiPortSwitch  DataPortForDefault=Additional data port  DiagnosticForDefault=None
  Mux1 : Mux  Inputs=2
  Reshape : Reshape  OutputDimensionality=Customize  OutputDimensions=[16,1]
  Standby : Constant  Value=ones(8,1)*1150  VectorParams1D=off  OutDataTypeStr=uint16
  cmd_out : Outport
  wires:
  Disarm/1 -> Multiport Switch/5, Multiport Switch/2
  Reshape/1 -> cmd_out/1
  Constant/1 -> Mux1/2
  Standby/1 -> Multiport Switch/3
  Mux1/1 -> Reshape/1
  status/1 -> Multiport Switch/1
  Multiport Switch/1 -> Mux1/1
  cmd_in/1 -> Multiport Switch/4

== system Controller/Controller/Control_Allocation/Octocopter_+/throttle_mapping ==
  theust_cmd : Inport
  Constant1 : Constant  Value=1000  OutDataTypeStr=uint32
  Data Type Conversion : DataTypeConversion  OutDataTypeStr=uint16
  Gain1 : Gain  Gain=1000  OutDataTypeStr=uint32
  Saturation : Saturate  UpperLimit=1  LowerLimit=0
  Sum : Sum  Inputs=|++
  Sum1 : Sum  Inputs=|++
  hover_throttle : Constant  Value=CONTROL_PARAM.HOVER_THRO  OutDataTypeStr=Inherit: Inherit via back propagation
  throttle_cmd : Outport
  wires:
  theust_cmd/1 -> Sum/1
  Sum/1 -> Saturation/1
  hover_throttle/1 -> Sum/2
  Gain1/1 -> Sum1/1
  Constant1/1 -> Sum1/2
  Data Type Conversion/1 -> throttle_cmd/1
  Saturation/1 -> Gain1/1
  Sum1/1 -> Data Type Conversion/1

== system Controller/Controller/Control_Allocation/Octocopter_x/Signal_Select ==
  note: mode:
      | 0: Unknown
      | 1: Mission
      | 2: Position
      | 3: Altitude Hold
      | 4: Manual Mode
      | 5: Acro Mode
  throttle_cmd_in : Inport
  FMS_Out : Inport  Port=2
  Bus Selector1 : BusSelector  OutputSignals=throttle_cmd,ctrl_mode
  Compare To Constant : simulink/Logic and Bit Operations/Compare To Constant  relop===  const=uint8([ControlMode.Manual, ControlMode.Acro, ControlMode.Stabilize])  OutDataTypeStr=boolean
  Compare To Constant1 : simulink/Logic and Bit Operations/Compare To Constant  relop===  const=uint8(ControlMode.Offboard)  OutDataTypeStr=boolean
  Logical Operator : Logic  Operator=OR  Inputs=1  AllPortsSameDT=off  OutDataTypeStr=boolean
  Offboard_Signal_Select : Subsystem
  Switch : Switch  Criteria=u2 > Threshold
  Switch1 : Switch  Criteria=u2 > Threshold
  throttle_cmd : Outport
  wires:
  Compare To Constant/1 -> Logical Operator/1
  FMS_Out/1 -> Offboard_Signal_Select/1(FMS_Out), Bus Selector1/1
  Bus Selector1/1 -> Switch/1  "<throttle_cmd>"
  Bus Selector1/2 -> Compare To Constant1/1, Compare To Constant/1  "<ctrl_mode>"
  Switch/1 -> throttle_cmd/1  "throttle_cmd"
  Logical Operator/1 -> Switch/2
  throttle_cmd_in/1 -> Offboard_Signal_Select/2(throttle_cmd_in), Switch1/3
  Compare To Constant1/1 -> Switch1/2
  Switch1/1 -> Switch/3
  Offboard_Signal_Select/1(throttle_cmd_out) -> Switch1/1

== system Controller/Controller/Control_Allocation/Octocopter_x/actuator_cmd_routing ==
  cmd_in : Inport
  status : Inport  Port=2
  Constant : Constant  Value=zeros(8,1)  VectorParams1D=off  OutDataTypeStr=uint16
  Disarm : Constant  Value=ones(8,1)*1000  VectorParams1D=off  OutDataTypeStr=uint16
  Multiport Switch : MultiPortSwitch  DataPortForDefault=Additional data port  DiagnosticForDefault=None
  Mux1 : Mux  Inputs=2
  Reshape : Reshape  OutputDimensionality=Customize  OutputDimensions=[16,1]
  Standby : Constant  Value=ones(8,1)*1150  VectorParams1D=off  OutDataTypeStr=uint16
  cmd_out : Outport
  wires:
  Disarm/1 -> Multiport Switch/5, Multiport Switch/2
  Reshape/1 -> cmd_out/1
  Constant/1 -> Mux1/2
  Standby/1 -> Multiport Switch/3
  Mux1/1 -> Reshape/1
  status/1 -> Multiport Switch/1
  Multiport Switch/1 -> Mux1/1
  cmd_in/1 -> Multiport Switch/4

== system Controller/Controller/Control_Allocation/Octocopter_x/throttle_mapping ==
  theust_cmd : Inport
  Constant1 : Constant  Value=1000  OutDataTypeStr=uint32
  Data Type Conversion : DataTypeConversion  OutDataTypeStr=uint16
  Gain1 : Gain  Gain=1000  OutDataTypeStr=uint32
  Saturation : Saturate  UpperLimit=1  LowerLimit=0
  Sum : Sum  Inputs=|++
  Sum1 : Sum  Inputs=|++
  hover_throttle : Constant  Value=CONTROL_PARAM.HOVER_THRO  OutDataTypeStr=Inherit: Inherit via back propagation
  throttle_cmd : Outport
  wires:
  theust_cmd/1 -> Sum/1
  Sum/1 -> Saturation/1
  hover_throttle/1 -> Sum/2
  Gain1/1 -> Sum1/1
  Constant1/1 -> Sum1/2
  Data Type Conversion/1 -> throttle_cmd/1
  Saturation/1 -> Gain1/1
  Sum1/1 -> Data Type Conversion/1

== system Controller/Controller/Control_Allocation/Quadcopter_+/Signal_Select ==
  note: mode:
      | 0: Unknown
      | 1: Mission
      | 2: Position
      | 3: Altitude Hold
      | 4: Manual Mode
      | 5: Acro Mode
  throttle_cmd_in : Inport
  FMS_Out : Inport  Port=2
  Bus Selector1 : BusSelector  OutputSignals=throttle_cmd,ctrl_mode
  Compare To Constant : simulink/Logic and Bit Operations/Compare To Constant  relop===  const=uint8([ControlMode.Manual, ControlMode.Acro, ControlMode.Stabilize])  OutDataTypeStr=boolean
  Compare To Constant1 : simulink/Logic and Bit Operations/Compare To Constant  relop===  const=uint8(ControlMode.Offboard)  OutDataTypeStr=boolean
  Logical Operator : Logic  Operator=OR  Inputs=1  AllPortsSameDT=off  OutDataTypeStr=boolean
  Offboard_Signal_Select : Subsystem
  Switch : Switch  Criteria=u2 > Threshold
  Switch1 : Switch  Criteria=u2 > Threshold
  throttle_cmd : Outport
  wires:
  Compare To Constant/1 -> Logical Operator/1
  FMS_Out/1 -> Offboard_Signal_Select/1(FMS_Out), Bus Selector1/1
  Bus Selector1/1 -> Switch/1  "<throttle_cmd>"
  Bus Selector1/2 -> Compare To Constant1/1, Compare To Constant/1  "<ctrl_mode>"
  Switch/1 -> throttle_cmd/1  "throttle_cmd"
  Logical Operator/1 -> Switch/2
  throttle_cmd_in/1 -> Offboard_Signal_Select/2(throttle_cmd_in), Switch1/3
  Compare To Constant1/1 -> Switch1/2
  Switch1/1 -> Switch/3
  Offboard_Signal_Select/1(throttle_cmd_out) -> Switch1/1

== system Controller/Controller/Control_Allocation/Quadcopter_+/actuator_cmd_routing ==
  cmd_in : Inport
  status : Inport  Port=2
  Constant : Constant  Value=zeros(12,1)  VectorParams1D=off  OutDataTypeStr=uint16
  Disarm : Constant  Value=ones(4,1)*1000  VectorParams1D=off  OutDataTypeStr=uint16
  Multiport Switch : MultiPortSwitch  DataPortForDefault=Additional data port  DiagnosticForDefault=None
  Mux1 : Mux  Inputs=2
  Reshape : Reshape  OutputDimensionality=Customize  OutputDimensions=[16,1]
  Standby : Constant  Value=ones(4,1)*1150  VectorParams1D=off  OutDataTypeStr=uint16
  cmd_out : Outport
  wires:
  Disarm/1 -> Multiport Switch/5, Multiport Switch/2
  Reshape/1 -> cmd_out/1
  Constant/1 -> Mux1/2
  Standby/1 -> Multiport Switch/3
  Mux1/1 -> Reshape/1
  status/1 -> Multiport Switch/1
  Multiport Switch/1 -> Mux1/1
  cmd_in/1 -> Multiport Switch/4

== system Controller/Controller/Control_Allocation/Quadcopter_+/throttle_mapping ==
  theust_cmd : Inport
  Constant1 : Constant  Value=1000  OutDataTypeStr=uint32
  Data Type Conversion : DataTypeConversion  OutDataTypeStr=uint16
  Gain1 : Gain  Gain=1000  OutDataTypeStr=uint32
  Saturation : Saturate  UpperLimit=1  LowerLimit=0
  Sum : Sum  Inputs=|++
  Sum1 : Sum  Inputs=|++
  hover_throttle : Constant  Value=CONTROL_PARAM.HOVER_THRO  OutDataTypeStr=Inherit: Inherit via back propagation
  throttle_cmd : Outport
  wires:
  theust_cmd/1 -> Sum/1
  Sum/1 -> Saturation/1
  hover_throttle/1 -> Sum/2
  Gain1/1 -> Sum1/1
  Constant1/1 -> Sum1/2
  Data Type Conversion/1 -> throttle_cmd/1
  Saturation/1 -> Gain1/1
  Sum1/1 -> Data Type Conversion/1

== system Controller/Controller/Control_Allocation/Quadcopter_x/Signal_Select ==
  note: mode:
      | 0: Unknown
      | 1: Mission
      | 2: Position
      | 3: Altitude Hold
      | 4: Manual Mode
      | 5: Acro Mode
  throttle_cmd_in : Inport
  FMS_Out : Inport  Port=2
  Bus Selector1 : BusSelector  OutputSignals=throttle_cmd,ctrl_mode
  Compare To Constant : simulink/Logic and Bit Operations/Compare To Constant  relop===  const=uint8([ControlMode.Manual, ControlMode.Acro, ControlMode.Stabilize])  OutDataTypeStr=boolean
  Compare To Constant1 : simulink/Logic and Bit Operations/Compare To Constant  relop===  const=uint8(ControlMode.Offboard)  OutDataTypeStr=boolean
  Logical Operator : Logic  Operator=OR  Inputs=1  AllPortsSameDT=off  OutDataTypeStr=boolean
  Offboard_Signal_Select : Subsystem
  Switch : Switch  Criteria=u2 > Threshold
  Switch1 : Switch  Criteria=u2 > Threshold
  throttle_cmd : Outport
  wires:
  Compare To Constant/1 -> Logical Operator/1
  FMS_Out/1 -> Offboard_Signal_Select/1(FMS_Out), Bus Selector1/1
  Bus Selector1/1 -> Switch/1  "<throttle_cmd>"
  Bus Selector1/2 -> Compare To Constant1/1, Compare To Constant/1  "<ctrl_mode>"
  Switch/1 -> throttle_cmd/1  "throttle_cmd"
  Logical Operator/1 -> Switch/2
  throttle_cmd_in/1 -> Offboard_Signal_Select/2(throttle_cmd_in), Switch1/3
  Compare To Constant1/1 -> Switch1/2
  Switch1/1 -> Switch/3
  Offboard_Signal_Select/1(throttle_cmd_out) -> Switch1/1

== system Controller/Controller/Control_Allocation/Quadcopter_x/actuator_cmd_routing ==
  cmd_in : Inport
  status : Inport  Port=2
  Constant : Constant  Value=zeros(12,1)  VectorParams1D=off  OutDataTypeStr=uint16
  Disarm : Constant  Value=ones(4,1)*1000  VectorParams1D=off  OutDataTypeStr=uint16
  Multiport Switch : MultiPortSwitch  DataPortForDefault=Additional data port  DiagnosticForDefault=None
  Mux1 : Mux  Inputs=2
  Reshape : Reshape  OutputDimensionality=Customize  OutputDimensions=[16,1]
  Standby : Constant  Value=ones(4,1)*1150  VectorParams1D=off  OutDataTypeStr=uint16
  cmd_out : Outport
  wires:
  Disarm/1 -> Multiport Switch/5, Multiport Switch/2
  Reshape/1 -> cmd_out/1
  Constant/1 -> Mux1/2
  Standby/1 -> Multiport Switch/3
  Mux1/1 -> Reshape/1
  status/1 -> Multiport Switch/1
  Multiport Switch/1 -> Mux1/1
  cmd_in/1 -> Multiport Switch/4

== system Controller/Controller/Control_Allocation/Quadcopter_x/throttle_mapping ==
  theust_cmd : Inport
  Constant1 : Constant  Value=1000  OutDataTypeStr=uint32
  Data Type Conversion : DataTypeConversion  OutDataTypeStr=uint16
  Gain1 : Gain  Gain=1000  OutDataTypeStr=uint32
  Saturation : Saturate  UpperLimit=1  LowerLimit=0
  Sum : Sum  Inputs=|++
  Sum1 : Sum  Inputs=|++
  hover_throttle : Constant  Value=CONTROL_PARAM.HOVER_THRO  OutDataTypeStr=Inherit: Inherit via back propagation
  throttle_cmd : Outport
  wires:
  theust_cmd/1 -> Sum/1
  Sum/1 -> Saturation/1
  hover_throttle/1 -> Sum/2
  Gain1/1 -> Sum1/1
  Constant1/1 -> Sum1/2
  Data Type Conversion/1 -> throttle_cmd/1
  Saturation/1 -> Gain1/1
  Sum1/1 -> Data Type Conversion/1

== system Controller/Controller/Horizontal_Control/Attitude_Controller/Inner_Loop ==
  euler_rate_cmd_radPs : Inport
  INS_Out : Inport  Port=2
  FMS_Out : Inport  Port=3
  Bus Selector : BusSelector  OutputSignals=reset
  Rate_Controller : Subsystem
  Signal_Convert : Subsystem
  Signal_Select : Subsystem
  rate_dot_cmd_B : Outport
  wires:
  euler_rate_cmd_radPs/1 -> Signal_Convert/2(euler_rate_cmd)
  Signal_Select/1(out) -> Rate_Controller/1(rate_cmd_radPs)
  Rate_Controller/1(rate_dot_cmd_B) -> rate_dot_cmd_B/1
  Bus Selector/1 -> Rate_Controller/3(reset)  "<reset>"
  INS_Out/1 -> Signal_Convert/3(INS_Out), Rate_Controller/2(INS_Out)
  FMS_Out/1 -> Signal_Convert/1(FMS_Out), Bus Selector/1, Signal_Select/1(FMS_Out)
  Signal_Convert/1(rate_cmd_radPs) -> Signal_Select/2(rate_cmd_radPs)

== system Controller/Controller/Horizontal_Control/Attitude_Controller/Outter_Loop ==
  att_cmd_rad : Inport
  INS_Out : Inport  Port=2
  FMS_Out : Inport  Port=3
  Attitude_Controller : Subsystem
  Signal_Select : Subsystem
  euler_rate_cmd_radPs : Outport
  wires:
  Signal_Select/1(out) -> Attitude_Controller/1(att_cmd_rad)
  FMS_Out/1 -> Signal_Select/2(FMS_Out)
  INS_Out/1 -> Attitude_Controller/2(INS_Out)
  Attitude_Controller/1(euler_rate_cmd_radPs) -> euler_rate_cmd_radPs/1
  att_cmd_rad/1 -> Signal_Select/1(att_cmd_rad)

== system Controller/Controller/Horizontal_Control/Velocity_Controller/Accel_to_Attitude_CMD ==
  note: Gain to resist
      | air drag
  accel_cmd_C_mPs2 : Inport
  Atan : Trigonometry  Operator=atan
  Divide : Product  Inputs=*/
  Gain1 : Gain  Gain=-1
  Mux : Mux  Inputs=2
  Saturation : Saturate  UpperLimit=CONTROL_PARAM.ROLL_PITCH_CMD_LIM  LowerLimit=-CONTROL_PARAM.ROLL_PITCH_CMD_LIM
  Selector : Selector  InputPortWidth=2  IndexOptions=Index vector (dialog)  Indices=1  OutputSizes=1
  Selector1 : Selector  InputPortWidth=2  IndexOptions=Index vector (dialog)  Indices=2  OutputSizes=1
  g : Constant  Value=9.8055  OutDataTypeStr=single
  gain : Gain  Gain=1.1
  att_cmd_B_rad : Outport
  wires:
  Mux/1 -> gain/1
  gain/1 -> Divide/1
  Atan/1 -> Saturation/1
  g/1 -> Divide/2
  Divide/1 -> Atan/1
  Selector/1 -> Gain1/1
  Selector1/1 -> Mux/1
  accel_cmd_C_mPs2/1 -> Selector/1, Selector1/1
  Gain1/1 -> Mux/2
  Saturation/1 -> att_cmd_B_rad/1

== system Controller/Controller/Horizontal_Control/Velocity_Controller/Error ==
  INS_Out : Inport
  FMS_Out : Inport  Port=2
  Bus Selector : BusSelector  OutputSignals=u_cmd,v_cmd,mode
  Bus_Select : Subsystem
  Compare To Constant : simulink/Logic and Bit Operations/Compare To Constant  relop=>=  const=uint8(PilotMode.Position)  OutDataTypeStr=boolean
  Data Type Conversion : DataTypeConversion  OutDataTypeStr=single
  Multiply : Product
  Mux : Mux  Inputs=2
  Sum : Sum  Inputs=|+-
  Switch : Switch  Criteria=u2 > Threshold
  TD : Subsystem
  uv_err_C_mPs : Outport
  wires:
  Sum/1 -> Multiply/2  "uv_error_C_mPs"
  FMS_Out/1 -> Bus Selector/1
  INS_Out/1 -> Bus_Select/1(INS_Out)
  Bus Selector/1 -> Mux/1  "<u_cmd>"
  Bus Selector/2 -> Mux/2  "<v_cmd>"
  TD/1(v1) -> Sum/1  "uv_cmd_C_mPs"
  Compare To Constant/1 -> Data Type Conversion/1, Switch/2
  Bus_Select/1(uv_est_C_mPs) -> Switch/3, Sum/2  "uv_est_C_mPs"
  Bus Selector/3 -> Compare To Constant/1  "<mode>"
  Mux/1 -> Switch/1
  Switch/1 -> TD/1(v)
  Multiply/1 -> uv_err_C_mPs/1  "uv_error_C_mPs"
  Data Type Conversion/1 -> Multiply/1

== system Controller/Controller/Horizontal_Control/Velocity_Controller/PID_Controller ==
  uv_err_C_mPs : Inport
  reset : Inport  Port=2
  Add : Sum  Inputs=+++
  D_Control : Subsystem  mask{kd=CONTROL_PARAM.VEL_XY_D, max_d=CONTROL_PARAM.VEL_XY_D_MAX, min_d=CONTROL_PARAM.VEL_XY_D_MIN}
  I_Control : Subsystem  mask{ki=CONTROL_PARAM.VEL_XY_I, max_i=CONTROL_PARAM.VEL_XY_I_MAX, min_i=CONTROL_PARAM.VEL_XY_I_MIN}
  P_Control : Subsystem  mask{kp=CONTROL_PARAM.VEL_XY_P}
  accel_cmd_C : Outport
  wires:
  uv_err_C_mPs/1 -> P_Control/1(err), I_Control/1(err), D_Control/1(err)
  reset/1 -> I_Control/2(reset), D_Control/2(reset)
  P_Control/1(p_out) -> Add/1  "accel_p_out"
  I_Control/1(i_out) -> Add/2  "accel_i_out"
  D_Control/1(d_out) -> Add/3  "accel_d_out"
  Add/1 -> accel_cmd_C/1

== system Controller/Controller/Horizontal_Control/Velocity_Controller/Signal_Select ==
  acc_cmd_in : Inport
  FMS_Out : Inport  Port=2
  Bus Selector : BusSelector  OutputSignals=ctrl_mode
  Offboard : simulink/Logic and Bit Operations/Compare To Constant  relop===  const=uint8(ControlMode.Offboard)  OutDataTypeStr=boolean
  Offboard_Signal_Select : Subsystem
  Switch : Switch  Criteria=u2 > Threshold
  acc_cmd_out : Outport
  wires:
  FMS_Out/1 -> Offboard_Signal_Select/1(FMS_Out), Bus Selector/1
  Bus Selector/1 -> Offboard/1  "<ctrl_mode>"
  Offboard/1 -> Switch/2
  Switch/1 -> acc_cmd_out/1
  acc_cmd_in/1 -> Offboard_Signal_Select/2(acc_cmd_in), Switch/3
  Offboard_Signal_Select/1(acc_cmd) -> Switch/1

== system Controller/Controller/Vertical_Control/Veloxity_Z_Controller/Boosted_Throttle ==
  thrust_cmd : Inport
  INS_Out : Inport  Port=2
  Bus Selector : BusSelector  OutputSignals=phi,theta
  Constant : Constant  OutDataTypeStr=single
  Cos : Trigonometry  Operator=cos
  Cos1 : Trigonometry  Operator=cos
  Divide : Product  Inputs=*/
  Gain : Gain  Gain=2
  Multiply : Product
  Multiply1 : Product  Inputs=3
  Saturation : Saturate  UpperLimit=1  LowerLimit=0
  Saturation1 : Saturate  UpperLimit=1  LowerLimit=0.5
  boosted_thrust : Outport
  wires:
  INS_Out/1 -> Bus Selector/1
  Bus Selector/1 -> Cos/1  "<phi>"
  Bus Selector/2 -> Cos1/1  "<theta>"
  Cos/1 -> Multiply/1
  Cos1/1 -> Multiply/2
  Multiply/1 -> Saturation1/1, Gain/1
  Gain/1 -> Saturation/1
  Saturation/1 -> Multiply1/3  "inverted_factor"
  Constant/1 -> Divide/1
  Divide/1 -> Multiply1/2  "boost_factor"
  Saturation1/1 -> Divide/2
  thrust_cmd/1 -> Multiply1/1
  Multiply1/1 -> boosted_thrust/1
